simulink model "NES2"  (R2019a)
settings: Solver=VariableStepAuto  StartTime=0.0  StopTime=10.0  RelTol=1e-3
InitFcn:
  | init
values from neighbouring files (symbols this model uses):
  c_ij = [c1,c2,c3,c4]    [C_ij.m]    (also in C_ij1.m = double(c_ij); Main.m = C_ij2_coef(c_2dot); Vafaei.m = C_ij2_coef(c_2dot))
  cdot = Cdot_coef(c_2dot)    [Main.m]    (also in Vafaei.m)
  dispturb = disturbance_coef(c_2dot)    [Main.m]    (also in Vafaei.m)
settings Model: Creator=NegarPajooh  LastModifiedBy=NegarPajooh

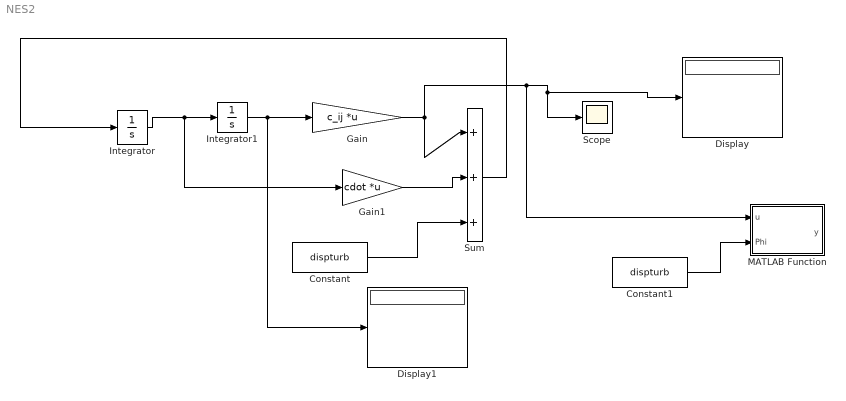
== system NES2 ==
  Constant : Constant  Value=dispturb
  Constant1 : Constant  Value=dispturb
  Display : Display
  Display1 : Display
  Gain : Gain  Gain=c_ij  Multiplication=Matrix(K*u) (u vector)
  Gain1 : Gain  Gain=cdot  Multiplication=Matrix(K*u) (u vector)
  Integrator : Integrator
  Integrator1 : Integrator
  MATLAB Function : MATLAB Function  TreatAsAtomicUnit=on
  Scope : Scope
  Sum : Sum  Inputs=|+++
  wires:
  Integrator/1 -> Gain1/1, Integrator1/1
  Integrator1/1 -> Display1/1, Gain/1
  Gain/1 -> MATLAB Function/1(u), Display/1, Scope/1, Sum/1
  Gain1/1 -> Sum/2
  Sum/1 -> Integrator/1
  Constant/1 -> Sum/3
  Constant1/1 -> MATLAB Function/2(Phi)

== matlab function NES2/MATLAB Function ==
  data: u input; y output; Phi input
function y = fcn(u,Phi)

y = u;
